simulink model "CM010A_GmT1xxMcuCfg"  (R2013b)
settings: Solver=FixedStepDiscrete  SolverMode=SingleTasking  StartTime=0.0  StopTime=0.05  RelTol=1e-3
undefined symbols (not defined in the file): BATTVLTGSCAGFAC_ULS_F32, BATTVLTGSWD1SCAGFAC_ULS_F32, BATTVLTGSWD2SCAGFAC_ULS_F32, sigbuilder_block
libraries: CM010A_GmT1xxMcuCfg_ModelLibrary x68, simulink x31
(part 3 of 3)

== system CM010A_GmT1xxMcuCfg/GmT1xxMcuCfg/GmT1xxMcuCfgPer1/CopyRight2 ==

== system CM010A_GmT1xxMcuCfg/GmT1xxMcuCfg/GmT1xxMcuCfgPer2/CopyRight2 ==

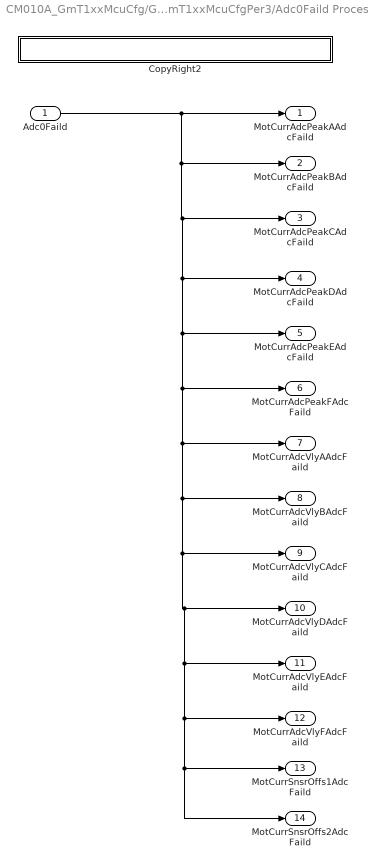
== system CM010A_GmT1xxMcuCfg/GmT1xxMcuCfg/GmT1xxMcuCfgPer3/Adc0Faild Processing ==
  Adc0Faild : Inport
  CopyRight2 : Subsystem  Description=|  mask(Copyright Information){none=on}
      | Copyright info block.                                               
      |                                                                     
      | Place copyright information at the top of every subsystem in design.
      mask prompts: none "No parameters"
      mask help: Place copyright information at the top of every subsystem in design.
      mask Display:
      | NxtrConf = 'Nexteer Confidential';
      | 
      | sys = bdroot; %handle for the current model ("system")
      | first = get_param(sys,'Created');
      | first = first(end-3:end);  %year is last four digits
      | 
      | last = get_param(sys,'LastModifiedDate');
      | if isempty(last)
      |     last = datestr(now,'yyyy');
      | else
      |     last = last(end-3:end);
      | end
      | 
      | if strcmp(first,last)
      |     fprintf('%s -- Copyright %s Nexteer',NxtrConf,first)
      | else
      |     fprintf('%s -- %s%s- %s Nexteer',NxtrConf,char(169),first,last)
      | end
  MotCurrAdcPeakAAdcFaild : Outport
  MotCurrAdcPeakBAdcFaild : Outport  Port=2
  MotCurrAdcPeakCAdcFaild : Outport  Port=3
  MotCurrAdcPeakDAdcFaild : Outport  Port=4
  MotCurrAdcPeakEAdcFaild : Outport  Port=5
  MotCurrAdcPeakFAdcFaild : Outport  Port=6
  MotCurrAdcVlyAAdcFaild : Outport  Port=7
  MotCurrAdcVlyBAdcFaild : Outport  Port=8
  MotCurrAdcVlyCAdcFaild : Outport  Port=9
  MotCurrAdcVlyDAdcFaild : Outport  Port=10
  MotCurrAdcVlyEAdcFaild : Outport  Port=11
  MotCurrAdcVlyFAdcFaild : Outport  Port=12
  MotCurrSnsrOffs1AdcFaild : Outport  Port=13
  MotCurrSnsrOffs2AdcFaild : Outport  Port=14
  wires:
  Adc0Faild/1 -> MotCurrSnsrOffs2AdcFaild/1, MotCurrSnsrOffs1AdcFaild/1, MotCurrAdcVlyFAdcFaild/1, MotCurrAdcVlyEAdcFaild/1, MotCurrAdcVlyDAdcFaild/1, MotCurrAdcVlyCAdcFaild/1, MotCurrAdcVlyBAdcFaild/1, MotCurrAdcVlyAAdcFaild/1, MotCurrAdcPeakFAdcFaild/1, MotCurrAdcPeakEAdcFaild/1, MotCurrAdcPeakDAdcFaild/1, MotCurrAdcPeakCAdcFaild/1, MotCurrAdcPeakBAdcFaild/1, MotCurrAdcPeakAAdcFaild/1

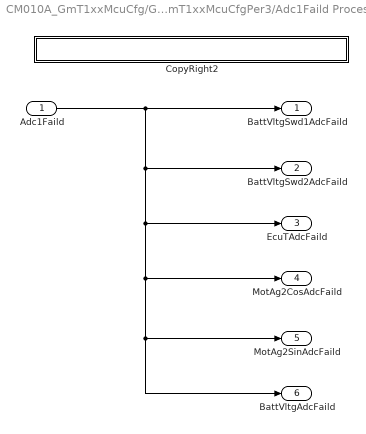
== system CM010A_GmT1xxMcuCfg/GmT1xxMcuCfg/GmT1xxMcuCfgPer3/Adc1Faild Processing ==
  Adc1Faild : Inport
  CopyRight2 : Subsystem  Description=|  mask(Copyright Information){none=on}
      | Copyright info block.                                               
      |                                                                     
      | Place copyright information at the top of every subsystem in design.
      mask prompts: none "No parameters"
      mask help: Place copyright information at the top of every subsystem in design.
      mask Display:
      | NxtrConf = 'Nexteer Confidential';
      | 
      | sys = bdroot; %handle for the current model ("system")
      | first = get_param(sys,'Created');
      | first = first(end-3:end);  %year is last four digits
      | 
      | last = get_param(sys,'LastModifiedDate');
      | if isempty(last)
      |     last = datestr(now,'yyyy');
      | else
      |     last = last(end-3:end);
      | end
      | 
      | if strcmp(first,last)
      |     fprintf('%s -- Copyright %s Nexteer',NxtrConf,first)
      | else
      |     fprintf('%s -- %s%s- %s Nexteer',NxtrConf,char(169),first,last)
      | end
  BattVltgSwd1AdcFaild : Outport
  BattVltgSwd2AdcFaild : Outport  Port=2
  EcuTAdcFaild : Outport  Port=3
  MotAg2CosAdcFaild : Outport  Port=4
  MotAg2SinAdcFaild : Outport  Port=5
  BattVltgAdcFaild : Outport  Port=6
  wires:
  Adc1Faild/1 -> MotAg2CosAdcFaild/1, BattVltgAdcFaild/1, MotAg2SinAdcFaild/1, EcuTAdcFaild/1, BattVltgSwd2AdcFaild/1, BattVltgSwd1AdcFaild/1

== system CM010A_GmT1xxMcuCfg/GmT1xxMcuCfg/GmT1xxMcuCfgPer3/CopyRight2 ==

== system CM010A_GmT1xxMcuCfg/GmT1xxMcuCfg/GmT1xxMcuCfgInit1/Register Initialization/CopyRight2 ==

== system CM010A_GmT1xxMcuCfg/GmT1xxMcuCfg/GmT1xxMcuCfgInit2/Process Initial Adc0/CopyRight2 ==

== system CM010A_GmT1xxMcuCfg/GmT1xxMcuCfg/GmT1xxMcuCfgInit2/Wait for ADC Conversion to Complete/CopyRight2 ==

== system CM010A_GmT1xxMcuCfg/GmT1xxMcuCfg/GmT1xxMcuCfgInit2/Wait for ADC Conversion to Complete/GetRefTmr1MicroSec32bit ==
  Ground : Ground
  RefTmr : Outport
  wires:
  Ground/1 -> RefTmr/1

== system CM010A_GmT1xxMcuCfg/GmT1xxMcuCfg/GmT1xxMcuCfgInit2/Wait for ADC Conversion to Complete/GetTiSpan1MicroSec32bit ==
  RefTmr : Inport
  Ground : Ground
  Terminator : Terminator
  TiSpan : Outport
  wires:
  Ground/1 -> TiSpan/1
  RefTmr/1 -> Terminator/1

== system CM010A_GmT1xxMcuCfg/GmT1xxMcuCfg/GmT1xxMcuCfgInit3/Process Initial Adc1/CopyRight2 ==

== system CM010A_GmT1xxMcuCfg/GmT1xxMcuCfg/GmT1xxMcuCfgPer3/Adc0Faild Processing/CopyRight2 ==

== system CM010A_GmT1xxMcuCfg/GmT1xxMcuCfg/GmT1xxMcuCfgPer3/Adc1Faild Processing/CopyRight2 ==
